simulink model "siso_4ch_teleop"  (R2021b)
settings: Solver=VariableStepAuto  StartTime=0.0  StopTime=10.0  RelTol=1e-3
values from neighbouring files (symbols this model uses):
  A = 1    [assignment1.m]
  As = 2.5    [assignment1.m]
  Be = 100    [assignment1.m]
  Bh = 1    [assignment1.m]
  Bm = 20*0.8    (= 16)    [assignment1.m]
  Bs = 4*Bm    (= 64)    [assignment1.m]
  Dh = 20*0.8    (= 16)    [assignment1.m]
  Dm = 5    [assignment1.m]
  Ds = 10    [assignment1.m]
  Fc = 1    [assignment1.m]
  Flp = 1    [assignment1.m]
  Jh = 1    [assignment1.m]
  Ke = 200    [assignment1.m]
  Kh = 0    [assignment1.m]
  Km = 10*1    (= 10)    [assignment1.m]
  Ks = 4*Km    (= 40)    [assignment1.m]
  Mm = 0.5    [assignment1.m]
  Ms = 2    [assignment1.m]
  Ph = 10*1    (= 10)    [assignment1.m]
  Ts = 0.001    [assignment1.m]
  xe = 1.5    [assignment1.m]
settings Model: Creator=buse  LastModifiedBy=buse

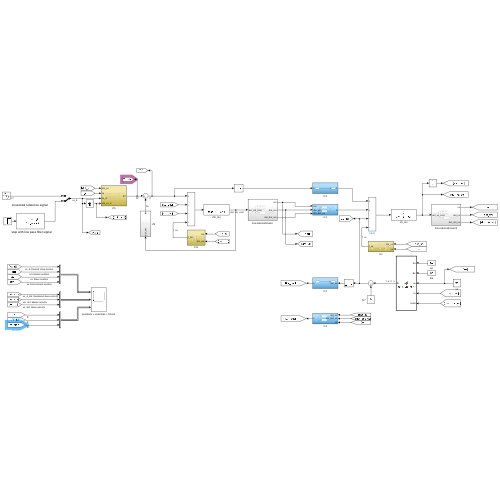
[thumbnail: Simulink's stored preview of the top-level diagram]
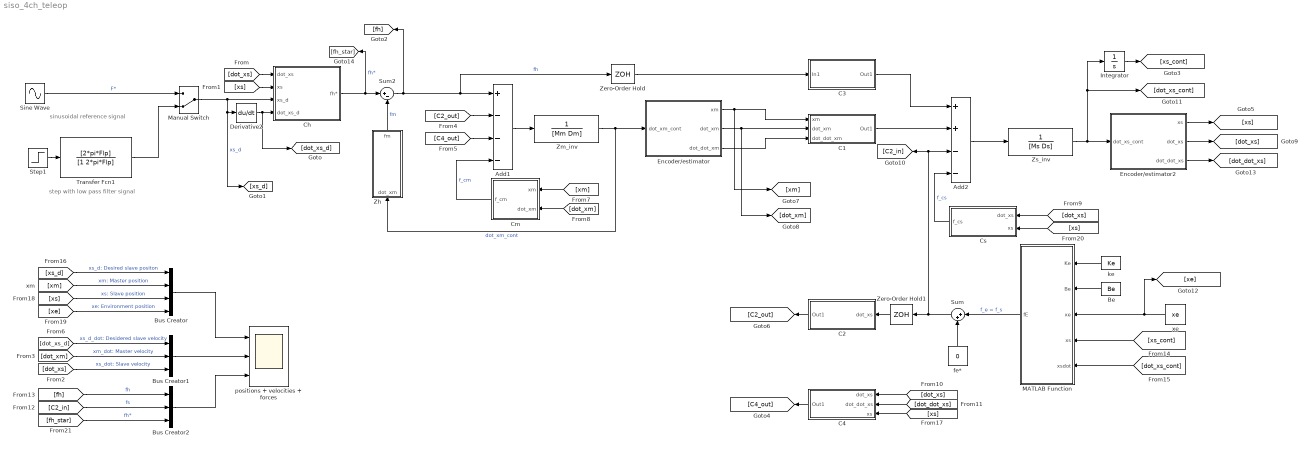
== system siso_4ch_teleop ==
  note: sinusoidal reference signal
  note: step with low pass filter signal
  Add1 : Sum  Inputs=+---
  Add2 : Sum  Inputs=++--
  Be : Constant  Value=Be
  Bus Creator : BusCreator  Inputs=4
  Bus Creator1 : BusCreator  Inputs=3
  Bus Creator2 : BusCreator  Inputs=3
  C1 : Subsystem
  C2 : Subsystem
  C3 : Subsystem
  C4 : Subsystem
  Ch : Subsystem
  Cm : Subsystem
  Cs : Subsystem
  Derivative2 : Derivative
  Encoder/estimator : Subsystem
  Encoder/estimator2 : Subsystem
  Integrator : Integrator
  MATLAB Function : MATLAB Function  TreatAsAtomicUnit=on
  Manual Switch : ManualSwitch  CurrentSetting=0
  Sine Wave : Sin  Amplitude=A  Frequency=Fc*2*pi  SampleTime=0
  Step1 : Step  After=As  SampleTime=0
  Sum : Sum  Inputs=|++
  Sum2 : Sum  Inputs=|+-
  Transfer Fcn1 : TransferFcn  Numerator=[2*pi*Flp]  Denominator=[1 2*pi*Flp]
  Zero-Order Hold : ZeroOrderHold  SampleTime=Ts
  Zero-Order Hold1 : ZeroOrderHold  SampleTime=Ts
  Zh : Subsystem
  Zm_inv : TransferFcn  Numerator=[0 1]  Denominator=[Mm Dm]
  Zs_inv : TransferFcn  Numerator=[0 1]  Denominator=[Ms Ds]
  fe* : Constant  Value=0
  ke : Constant  Value=Ke
  positions + velocities + forces : Scope  NumInputPorts=3
  xe : Constant  Value=xe
  wires:
  ke/1 -> MATLAB Function/1(Ke)
  xe/1 -> [xe], MATLAB Function/3(xe)
  Be/1 -> MATLAB Function/2(Be)
  Step1/1 -> Transfer Fcn1/1
  Zh/1(fm) -> Sum2/2  "fm"
  Manual Switch/1 -> Ch/3(xs_d), [xs_d], Derivative2/1  "xs_d"
  Sine Wave/1 -> Manual Switch/1  "F*"
  Ch/1(fh*) -> [fh_star], Sum2/1  "fh*"
  Transfer Fcn1/1 -> Manual Switch/2
  [dot_xs] -> Ch/1(dot_xs)
  [xs] -> Ch/2(xs)
  Sum2/1 -> [fh], Zero-Order Hold/1, Add1/1  "fh"
  [C2_out] -> Add1/2
  [C4_out] -> Add1/3
  Cm/1(f_cm) -> Add1/4  "f_cm"
  [xm] -> Cm/1(xm)
  [dot_xm] -> Cm/2(dot_xm)
  Add1/1 -> Zm_inv/1
  C1/1(Out1) -> Add2/2
  C3/1(Out1) -> Add2/1
  Zm_inv/1 -> Encoder/estimator/1(dot_xm_cont), Zh/1(dot_xm)  "dot_xm_cont"
  Add2/1 -> Zs_inv/1
  Cs/1(f_cs) -> Add2/4  "f_cs"
  Zs_inv/1 -> Integrator/1, [dot_xs_cont], Encoder/estimator2/1(dot_xs_cont)
  Encoder/estimator2/2(dot_xs) -> [dot_xs]
  Encoder/estimator2/1(xs) -> [xs]
  C2/1(Out1) -> [C2_out]
  MATLAB Function/1(fE) -> Sum/1  "f_e = f_s"
  fe*/1 -> Sum/2
  Sum/1 -> Add2/3, [C2_in], Zero-Order Hold1/1
  C4/1(Out1) -> [C4_out]
  Integrator/1 -> [xs_cont]
  [xs_cont] -> MATLAB Function/4(xs)
  [dot_xs_cont] -> MATLAB Function/5(xsdot)
  [xs_d] -> Bus Creator/1  "xs_d: Desired slave positon"
  [xm] -> Bus Creator/2  "xm: Master position"
  [xs] -> Bus Creator/3  "xs: Slave position"
  [xe] -> Bus Creator/4  "xe: Environment position"
  [dot_xs_d] -> Bus Creator1/1  "xs_d_dot: Desidered slave velocity"
  [dot_xm] -> Bus Creator1/2  "xm_dot: Master velocity"
  [dot_xs] -> Bus Creator1/3  "xs_dot: Slave velocity"
  [fh] -> Bus Creator2/1  "fh"
  [C2_in] -> Bus Creator2/2  "fs"
  Zero-Order Hold/1 -> C3/1(In1)
  Zero-Order Hold1/1 -> C2/1(dot_xs)
  Encoder/estimator2/3(dot_dot_xs) -> [dot_dot_xs]
  [dot_xs] -> Cs/1(dot_xs)
  [dot_xs] -> C4/1(dot_xs)
  [xs] -> C4/3(xs)
  [dot_dot_xs] -> C4/2(dot_dot_xs)
  Encoder/estimator/1(xm) -> [xm], C1/1(xm)
  Encoder/estimator/2(dot_xm) -> [dot_xm], C1/2(dot_xm)
  Encoder/estimator/3(dot_dot_xm) -> C1/3(dot_dot_xm)
  Bus Creator/1 -> positions + velocities + forces/1
  Bus Creator1/1 -> positions + velocities + forces/2
  Bus Creator2/1 -> positions + velocities + forces/3
  Derivative2/1 -> [dot_xs_d], Ch/4(dot_xs_d)
  [xs] -> Cs/2(xs)
  [fh_star] -> Bus Creator2/3  "fh*"

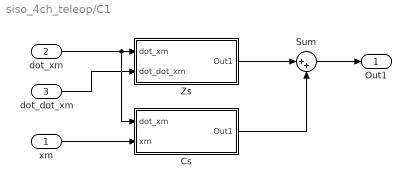
== system siso_4ch_teleop/C1 ==
  xm : Inport
  dot_xm : Inport  Port=2
  dot_dot_xm : Inport  Port=3
  Cs : Subsystem
  Sum : Sum  Inputs=|++
  Zs : Subsystem
  Out1 : Outport
  wires:
  dot_xm/1 -> Cs/1(dot_xm), Zs/1(dot_xm)
  Zs/1(Out1) -> Sum/1
  Cs/1(Out1) -> Sum/2
  Sum/1 -> Out1/1
  dot_dot_xm/1 -> Zs/2(dot_dot_xm)
  xm/1 -> Cs/2(xm)

== system siso_4ch_teleop/C2 ==
  dot_xs : Inport
  Out1 : Outport
  wires:
  dot_xs/1 -> Out1/1

== system siso_4ch_teleop/C3 ==
  In1 : Inport
  Out1 : Outport
  wires:
  In1/1 -> Out1/1

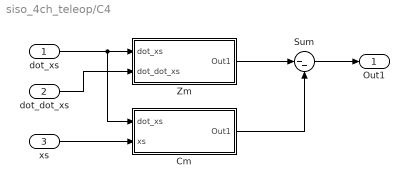
== system siso_4ch_teleop/C4 ==
  dot_xs : Inport
  dot_dot_xs : Inport  Port=2
  xs : Inport  Port=3
  Cm : Subsystem
  Sum : Sum  Inputs=|--
  Zm : Subsystem
  Out1 : Outport
  wires:
  dot_xs/1 -> Zm/1(dot_xs), Cm/1(dot_xs)
  Zm/1(Out1) -> Sum/1
  Cm/1(Out1) -> Sum/2
  Sum/1 -> Out1/1
  dot_dot_xs/1 -> Zm/2(dot_dot_xs)
  xs/1 -> Cm/2(xs)

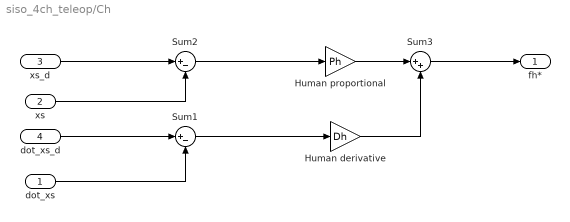
== system siso_4ch_teleop/Ch ==
  dot_xs : Inport
  xs : Inport  Port=2
  xs_d : Inport  Port=3
  dot_xs_d : Inport  Port=4
  Human derivative : Gain  Gain=Dh
  Human proportional : Gain  Gain=Ph
  Sum1 : Sum  Inputs=|+-
  Sum2 : Sum  Inputs=|+-
  Sum3 : Sum  Inputs=|++
  fh* : Outport
  wires:
  xs/1 -> Sum2/2
  dot_xs/1 -> Sum1/2
  Sum2/1 -> Human proportional/1
  Sum1/1 -> Human derivative/1
  Human derivative/1 -> Sum3/2
  Human proportional/1 -> Sum3/1
  Sum3/1 -> fh*/1
  xs_d/1 -> Sum2/1
  dot_xs_d/1 -> Sum1/1

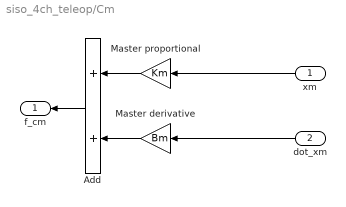
== system siso_4ch_teleop/Cm ==
  xm : Inport
  dot_xm : Inport  Port=2
  Add : Sum
  Master derivative : Gain  Gain=Bm
  Master proportional : Gain  Gain=Km
  f_cm : Outport
  wires:
  dot_xm/1 -> Master derivative/1
  xm/1 -> Master proportional/1
  Master proportional/1 -> Add/1
  Master derivative/1 -> Add/2
  Add/1 -> f_cm/1

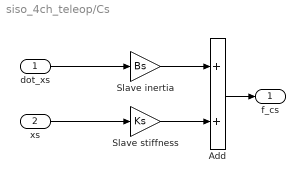
== system siso_4ch_teleop/Cs ==
  dot_xs : Inport
  xs : Inport  Port=2
  Add : Sum
  Slave inertia : Gain  Gain=Bs
  Slave stiffness : Gain  Gain=Ks
  f_cs : Outport
  wires:
  dot_xs/1 -> Slave inertia/1
  xs/1 -> Slave stiffness/1
  Slave stiffness/1 -> Add/2
  Slave inertia/1 -> Add/1
  Add/1 -> f_cs/1

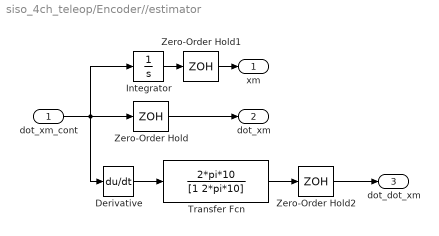
== system siso_4ch_teleop/Encoder//estimator ==
  dot_xm_cont : Inport
  Derivative : Derivative
  Integrator : Integrator
  Transfer Fcn : TransferFcn  Numerator=2*pi*10  Denominator=[1 2*pi*10]
  Zero-Order Hold : ZeroOrderHold  SampleTime=-1
  Zero-Order Hold1 : ZeroOrderHold  SampleTime=Ts
  Zero-Order Hold2 : ZeroOrderHold  SampleTime=Ts
  xm : Outport
  dot_xm : Outport  Port=2
  dot_dot_xm : Outport  Port=3
  wires:
  dot_xm_cont/1 -> Derivative/1, Integrator/1, Zero-Order Hold/1
  Integrator/1 -> Zero-Order Hold1/1
  Zero-Order Hold1/1 -> xm/1
  Zero-Order Hold/1 -> dot_xm/1
  Transfer Fcn/1 -> Zero-Order Hold2/1
  Derivative/1 -> Transfer Fcn/1
  Zero-Order Hold2/1 -> dot_dot_xm/1

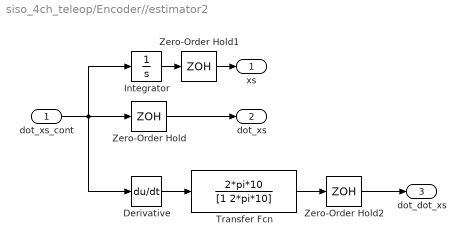
== system siso_4ch_teleop/Encoder//estimator2 ==
  dot_xs_cont : Inport
  Derivative : Derivative
  Integrator : Integrator
  Transfer Fcn : TransferFcn  Numerator=2*pi*10  Denominator=[1 2*pi*10]
  Zero-Order Hold : ZeroOrderHold  SampleTime=-1
  Zero-Order Hold1 : ZeroOrderHold  SampleTime=Ts
  Zero-Order Hold2 : ZeroOrderHold  SampleTime=Ts
  xs : Outport
  dot_xs : Outport  Port=2
  dot_dot_xs : Outport  Port=3
  wires:
  dot_xs_cont/1 -> Derivative/1, Integrator/1, Zero-Order Hold/1
  Zero-Order Hold/1 -> dot_xs/1
  Integrator/1 -> Zero-Order Hold1/1
  Zero-Order Hold1/1 -> xs/1
  Derivative/1 -> Transfer Fcn/1
  Transfer Fcn/1 -> Zero-Order Hold2/1
  Zero-Order Hold2/1 -> dot_dot_xs/1

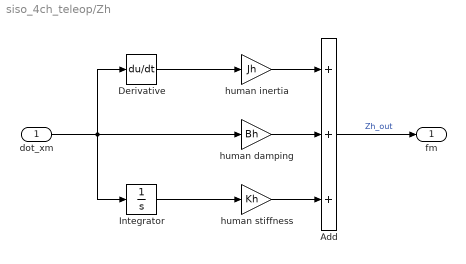
== system siso_4ch_teleop/Zh ==
  dot_xm : Inport
  Add : Sum  Inputs=+++
  Derivative : Derivative
  Integrator : Integrator
  human damping : Gain  Gain=Bh
  human inertia : Gain  Gain=Jh
  human stiffness : Gain  Gain=Kh
  fm : Outport
  wires:
  Add/1 -> fm/1  "Zh_out"
  dot_xm/1 -> Integrator/1, Derivative/1, human damping/1
  Derivative/1 -> human inertia/1
  Integrator/1 -> human stiffness/1
  human damping/1 -> Add/2
  human inertia/1 -> Add/1
  human stiffness/1 -> Add/3

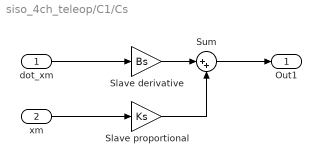
== system siso_4ch_teleop/C1/Cs ==
  dot_xm : Inport
  xm : Inport  Port=2
  Slave derivative : Gain  Gain=Bs
  Slave proportional : Gain  Gain=Ks
  Sum : Sum  Inputs=|++
  Out1 : Outport
  wires:
  dot_xm/1 -> Slave derivative/1
  xm/1 -> Slave proportional/1
  Slave derivative/1 -> Sum/1
  Slave proportional/1 -> Sum/2
  Sum/1 -> Out1/1

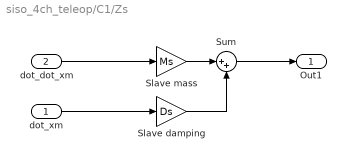
== system siso_4ch_teleop/C1/Zs ==
  dot_xm : Inport
  dot_dot_xm : Inport  Port=2
  Slave damping : Gain  Gain=Ds
  Slave mass : Gain  Gain=Ms
  Sum : Sum  Inputs=|++
  Out1 : Outport
  wires:
  dot_xm/1 -> Slave damping/1
  dot_dot_xm/1 -> Slave mass/1
  Slave mass/1 -> Sum/1
  Slave damping/1 -> Sum/2
  Sum/1 -> Out1/1

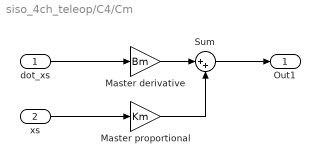
== system siso_4ch_teleop/C4/Cm ==
  dot_xs : Inport
  xs : Inport  Port=2
  Master derivative : Gain  Gain=Bm
  Master proportional : Gain  Gain=Km
  Sum : Sum  Inputs=|++
  Out1 : Outport
  wires:
  dot_xs/1 -> Master derivative/1
  xs/1 -> Master proportional/1
  Master derivative/1 -> Sum/1
  Master proportional/1 -> Sum/2
  Sum/1 -> Out1/1

== system siso_4ch_teleop/C4/Zm ==
  dot_xs : Inport
  dot_dot_xs : Inport  Port=2
  Master damping : Gain  Gain=Dm
  Master mass : Gain  Gain=Mm
  Sum : Sum  Inputs=|++
  Out1 : Outport
  wires:
  dot_xs/1 -> Master damping/1
  dot_dot_xs/1 -> Master mass/1
  Master mass/1 -> Sum/1
  Master damping/1 -> Sum/2
  Sum/1 -> Out1/1

== matlab function siso_4ch_teleop/MATLAB Function ==
  data: Ke input; fE output; Be input; xe input; xs input; xsdot input
function fE = environment(Ke, Be, xe, xs, xsdot)
    if xs > xe
        fE = Ke * (xs - xe) + Be * xsdot; % Plot both contributions Ke and Be
    else
        fE = 0;
    end
end
